simulink model "exercise10"  (R2017a)
settings: Solver=VariableStepAuto  StartTime=0.0  StopTime=30  RelTol=1e-3
settings Model: Creator=viktor  LastModifiedBy=viktor

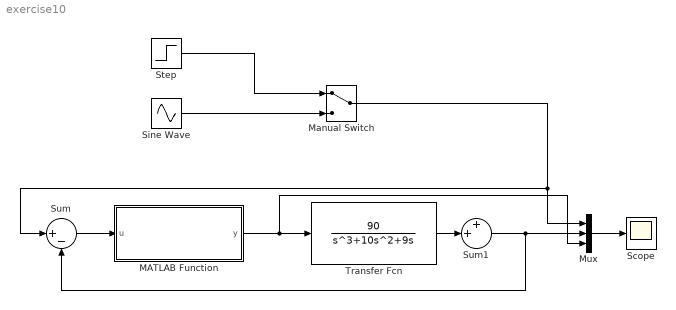
== system exercise10 ==
  MATLAB Function : MATLAB Function  TreatAsAtomicUnit=on
  Manual Switch : ManualSwitch
  Mux : Mux  Inputs=3
  Scope : Scope
  Sine Wave : Sin  Amplitude=.01  Frequency=3  SampleTime=0
  Step : Step  After=2  SampleTime=0
  Sum : Sum  Inputs=|+-
  Sum1 : Sum  Inputs=++|
  Transfer Fcn : TransferFcn  Numerator=[90]  Denominator=[1 10 9 0]
  wires:
  MATLAB Function/1(y) -> Mux/3, Transfer Fcn/1
  Sum/1 -> MATLAB Function/1(u)
  Mux/1 -> Scope/1
  Transfer Fcn/1 -> Sum1/2
  Sum1/1 -> Sum/2, Mux/2
  Sine Wave/1 -> Manual Switch/2
  Step/1 -> Manual Switch/1
  Manual Switch/1 -> Mux/1, Sum/1

== matlab function exercise10/MATLAB Function ==
  data: u input; y output
function y = relay_with_deadzone(u)
    if u <= -.2
        y = -1;
    elseif u >= .2
        y = 1;
    else
        y = 0;
    end
end
